simulink model "pathFollowingController_th"  (R2018b)
settings: Solver=VariableStepAuto  StartTime=0.0  StopTime=10.0  RelTol=1e-3
undefined symbols (not defined in the file or in its folder): chi_des, eul_ang, flow, pos, vel
libraries: pathFollowingController_cl x1
settings Model: Creator=jldanie5  LastModifiedBy=jldanie5

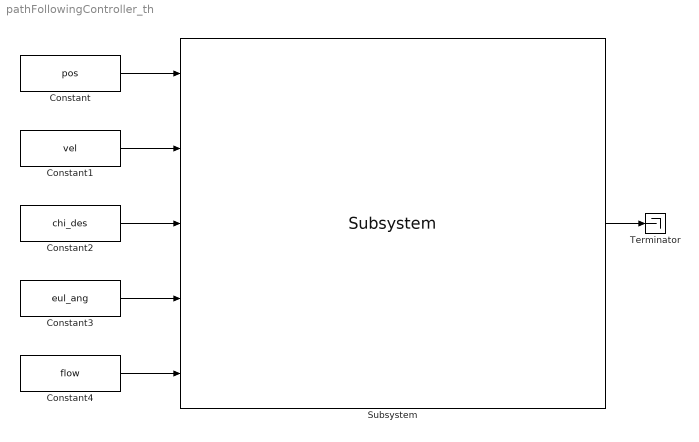
== system pathFollowingController_th ==
  Constant : Constant  Value=pos
  Constant1 : Constant  Value=vel
  Constant2 : Constant  Value=chi_des
  Constant3 : Constant  Value=eul_ang
  Constant4 : Constant  Value=flow
  Subsystem : pathFollowingController_cl/Subsystem  AoA_des=8  controlMat=controlmat  ctrlSigMax=controlmax
  Terminator : Terminator
  wires:
  Constant/1 -> Subsystem/1
  Constant1/1 -> Subsystem/2
  Constant2/1 -> Subsystem/3
  Constant3/1 -> Subsystem/4
  Constant4/1 -> Subsystem/5
  Subsystem/1 -> Terminator/1
